simulink model "Sensors_and_actuators_ball_and_plate"  (R2022b)
settings: Solver=ode1  StartTime=0.0  StopTime=Inf  FixedStep=0.001  RelTol=1e-3
PostLoadFcn:
  | , if any(exist('dsrtsu_mdlpostloadfcn', 'file') ~= 0), dsrtsu_mdlpostloadfcn('Execute', bdroot); end,
InitFcn:
  | , if any(exist('rtifpga_mdlclblib', 'file') ~= 0), rtifpga_mdlclblib('Init', bdroot); end,
values from neighbouring files (symbols this model uses):
  denc_mi = C.Denominator{:}    [main.m]
  numc_mi = C.Numerator{:}    [main.m]
libraries: rtiemclib x6, rtiethernetlib x3, rti1202lib_dac_class1 x3
(part 2 of 2)

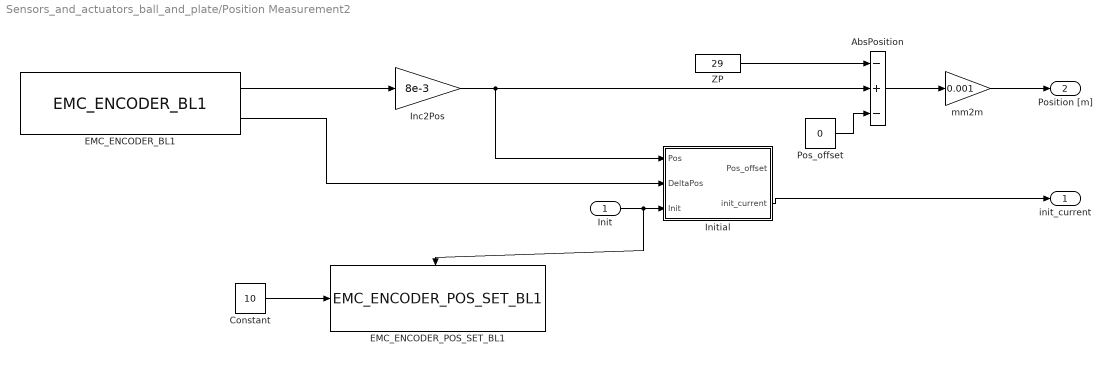
== system Sensors_and_actuators_ball_and_plate/Position Measurement2 ==
  Init : Inport
  AbsPosition : Sum  Inputs=-+-  SaturateOnIntegerOverflow=on
  Constant : Constant  Value=10
  EMC_ENCODER_BL1 : rtiemclib/EMC_ENCODER_BL1  DSProperties=struct('RTI',struct('Version',uint32(2),'BlockType',struct('isSLSource',uint8(1),'isSLSink',uint8(0),'isHWSource',uint8(1),'isHWSink',uint8(0),'isSetup',uint8(0),'isInline',uint8(1),'isNonInline',uint8(0),'isInterrupt',uint8(0),'isChannelwise',uint8(1)),'IOBoardType','DSEMC','UnitType','ENCODER','Identifier','ENCODER','DialogType','ML','BlockSet','RTIEMC','SlaveProcessor','NONE'))  RTIBlockInterface=struct('OutputPortsWidth',int32([1 1 1]),'OutputPortsActive',int32([1 1 0]),'OutputPortsName',{{'Position','Speed',['Index Detected']}},'OutputPortsDataType',{{'SS_DOUBLE','SS_DOUBLE','SS_BOOLEAN'}},'InitLevel',3,'IconTransparency','on','BlockDisplay',{{['EMC Encoder\nUnit: 3\nDIO class: 2\nPort: 1\nChannel: 5'],'center'}},'DialogFcn','rtiemcencodergui','BlockName',struct('Token',{{'EMC_ENCODER_BL1'}}))  RTIBlockParameters=struct('UnitNo',{{3,'OFF',[1 6]}},'DioClassNo',{{2,'OFF',[1 2]}},'PortNo',{{1,'OFF',[1 1]}},'ChannelNo',{{5,'OFF',[1 11]}},'HwSignalPin',{{['DIO1 ch1'],'OFF',[]}},'HwRefPin',{{'GND','OFF',[]}},'EnablePosMeasurement',{{1,'OFF',[0 1]}},'IndexSetMode',{{1,'OFF',[1 3]}},'EnableMinSpeed',{{0,'OFF',[0 1]}},'NumOfLines',{{'1024','OFF',[1 2097152]}},'InitAngleValue',{{'60','OFF',[0 359.99999]}},'IndexAngleValue',{{'0','OFF',[0 359.99999]}},'MinSpeedAngleValue',{{'45','OFF',[0.05 10000]}},'MinPosValue',{{'0','OFF',[-2097152 2097150.75]}},'MaxPosValue',{{'10000','OFF',[-2097151 2097151.75]}},'InitPosValue',{{'0','OFF',[-2097152 2097151.75]}},'IndexPosValue',{{'0','OFF',[-2097152 2097151.75]}},'MinSpeedPosValue',{{'100','OFF',[1 1000000]}},'IndexGateMode',{{0,'OFF',[0 1]}},'EnableNoiseFilter',{{0,'OFF',[0 1]}},'FilterInterval',{{'0','OFF',[0 0.01]}},'IndexDetectedOutPortMode',{{0,'OFF',[0 1]}},'BuildCheckAngleMeasurement',{{0,'OFF',[0 1]}},'BuildCheckAngleIndexMode',{{0,'OFF',[0 1]}},'BuildCheckPosIndexMode',{{0,'OFF',[0 1]}},'BuildCheckAngleMinSpeed',{{0,'OFF',[0 1]}},'BuildCheckPosMinSpeed',{{0,'OFF',[0 1]}},'TLCFileName',{{'rtiemcencoder','OFF',[]}})  RTISFcnParameters=struct('UnitNo','int32','DioClassNo','int32','PortNo','int32','ChannelNo','int32','EnablePosMeasurement','int32','IndexSetMode','int32','IndexDetectedOutPortMode','int32','EnableMinSpeed','int32','NumOfLines','uint32','InitAngleValue','double','IndexAngleValue','double','MinSpeedAngleValue','double','MinPosValue','double','MaxPosValue','double','InitPosValue','double','IndexPosValue','double','MinSpeedPosValue','double','IndexGateMode','int32','EnableNoiseFilter','int32','FilterInterval','double','TLCFileName','char')  RTIBlockParaDefault=struct('UnitNo',1,'DioClassNo',1,'PortNo',1,'ChannelNo',1,'HwSignalPin',['DIO1 ch1'],'HwRefPin','GND','EnablePosMeasurement',0,'IndexSetMode',1,'EnableMinSpeed',0,'NumOfLines',1024,'InitAngleValue',60,'IndexAngleValue',0,'MinSpeedAngleValue',45,'MinPosValue',0,'MaxPosValue',1023.75,'InitPosValue',0,'IndexPosValue',0,'MinSpeedPosValue',100,'IndexGateMode',0,'EnableNoiseFilter',0,'FilterInterval',0,'IndexDetectedOutPortMode',0,'BuildCheckAngleMeasurement',1,'BuildCheckAngleIndexMode',0,'BuildCheckPosIndexMode',0,'BuildCheckAngleMinSpeed',0,'BuildCheckPosMinSpeed',0,'TLCFileName','rtiemcencoder')
  EMC_ENCODER_POS_SET_BL1 : rtiemclib/EMC_ENCODER_POS_SET_BL1  DSProperties=struct('RTI',struct('Version',uint32(1),'BlockType',struct('isSLSource',uint8(0),'isSLSink',uint8(1),'isHWSource',uint8(0),'isHWSink',uint8(1),'isSetup',uint8(0),'isInline',uint8(1),'isNonInline',uint8(0),'isInterrupt',uint8(0),'isChannelwise',uint8(1)),'IOBoardType','DSEMC','UnitType','ENCODER','Identifier','ENCODERPOSSET','DialogType','ML','BlockSet','RTIEMC','SlaveProcessor','NONE'))  RTIBlockInterface=struct('InputPortsWidth',int32(1),'InputPortsActive',1,'InputPortsDataType',{{'SS_DOUBLE'}},'InputPortsName',{{'Position'}},'TriggerPort',{{'rising'}},'InitLevel',3,'IconTransparency','on','BlockDisplay',{{['EMC Encoder Position Set\nUnit: 3\nDIO class: 2\nPort: 1\nChannel: 5'],'center'}},'DialogFcn','rtiemcencoderpossetgui','BlockName',struct('Token',{{'EMC_ENCODER_POS_SET_BL1'}}))  RTIBlockParameters=struct('EncoderIdIndex',{{4,'OFF',[1 4]}},'UnitNo',{{3,'OFF',[]}},'DioClassNo',{{2,'OFF',[]}},'PortNo',{{1,'OFF',[]}},'ChannelNo',{{5,'OFF',[]}},'EnablePosMeasurement',{{1,'OFF',[]}},'NumOfLines',{{1024,'OFF',[]}},'TLCFileName',{{'rtiemcencoderposset','OFF',[]}})  RTISFcnParameters=struct('EncoderIdIndex','int32','UnitNo','int32','DioClassNo','int32','PortNo','int32','ChannelNo','int32','EnablePosMeasurement','int32','NumOfLines','int32','TLCFileName','char')  RTIBlockParaDefault=struct('EncoderIdIndex',1,'UnitNo',-1,'DioClassNo',-1,'PortNo',-1,'ChannelNo',-1,'EnablePosMeasurement',0,'NumOfLines',1024,'TLCFileName','rtiemcencoderposset')
  Inc2Pos : Gain  Gain=8e-3  SaturateOnIntegerOverflow=on  OutDataTypeStr=Inherit: Same as input  ParamDataTypeStr=Inherit: Same as input
  Initial : Subsystem
  Pos_offset : Constant  Value=0
  ZP : Constant  Value=29
  mm2m : Gain  Gain=0.001
  init_current : Outport  VectorParamsAs1DForOutWhenUnconnected=off
  Position [m] : Outport  Port=2  VectorParamsAs1DForOutWhenUnconnected=off
  wires:
  AbsPosition/1 -> mm2m/1
  Inc2Pos/1 -> Initial/1(Pos), AbsPosition/2
  Initial/2(init_current) -> init_current/1
  mm2m/1 -> Position [m]/1
  EMC_ENCODER_BL1/2 -> Initial/2(DeltaPos)
  ZP/1 -> AbsPosition/1
  Constant/1 -> EMC_ENCODER_POS_SET_BL1/1
  Init/1 -> Initial/3(Init), EMC_ENCODER_POS_SET_BL1/Trigger
  Pos_offset/1 -> AbsPosition/3
  EMC_ENCODER_BL1/1 -> Inc2Pos/1

== system Sensors_and_actuators_ball_and_plate/RTI Data ==
  RTI Data Store : Subsystem  Tag="struct('private',struct('version',struct('dsVer',uint32(2)),'access',struct('modified',['16-May-2023 15:23:02'],'type','Model','isPerm',1)),'public',struct('main',struct('data',[]),'sub',struct('name',{{'Sensors_and_actuators_ball_and_plate'}},'data',{{struct('TH',struct('thTaskInfo',struct('taskType',{'TIMER','HWINT','TMRINT','SWINT','GLINT'},'tasksNumOf',{1,0,0,0,0},'srcIds',{{'TIMERA'},{},{},{},{}},'taskNames',{{['Timer Task 1']},{},{},{},{}})),'th_tc',struct('dataType','TASK','taskGroupId','','taskGroupList',{{}},'taskSchedulingPolicy','FCFS','taskType','TIMER','blkh',-1,'srcId','TIMERA','srcSgnName',['Timer A interrupt'],'srcCpuName','','taskName',['Timer Task 1  [0.001] s'],'taskNameDisplayExt','','smplTime',0.001,'smplTimeOffs',0,'hasFixedPriority',0,'priority',1,'hasFixedOvc',0,'ovcType',1,'ovcMax',1),'tc_th',struct('dataType','TASK','taskGroupId','','taskGroupList',{{}},'taskSchedulingPolicy','FCFS','taskType','TIMER','blkh',-1,'srcId','TIMERA','srcSgnName',['Timer A interrupt'],'srcCpuName','','taskName',['Timer Task 1  [0.001] s'],'taskNameDisplayExt','','smplTime',0.001,'smplTimeOffs',0,'hasFixedPriority',0,'priority',1,'hasFixedOvc',0,'ovcType',1,'ovcMax',1))}})))"  mask(RTI_DATA_STORE){}
      mask help:
      | RTI Data Store Block. This block is used by RTI to store internal model dependent data. Deleting this block will result in data loss.
      |
      | NEVER DELETE, COPY, OR MODIFY THIS BLOCK!
      mask Help:
      | RTI Data Store Block. This block is used by RTI to store internal model dependent data. Deleting this block will result in data loss.
      | 
      | NEVER DELETE, COPY, OR MODIFY THIS BLOCK!
      mask Display: text(0.5, 0.5, ' ', 'HorizontalAlignment', 'center');

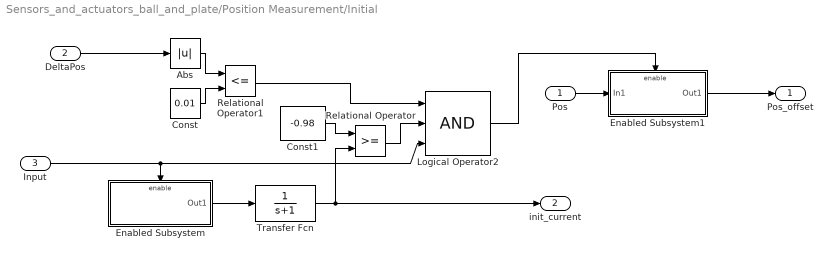
== system Sensors_and_actuators_ball_and_plate/Position Measurement/Initial ==
  Pos : Inport
  DeltaPos : Inport  Port=2
  Input : Inport  Port=3
  Abs : Abs
  Const : Constant  Value=0.01
  Const1 : Constant  Value=-0.98
  Enabled Subsystem : Subsystem  TreatAsAtomicUnit=on
  Enabled Subsystem1 : Subsystem  TreatAsAtomicUnit=on
  Logical Operator2 : Logic  Inputs=3  AllPortsSameDT=off
  Relational Operator : RelationalOperator  InputSameDT=off
  Relational Operator1 : RelationalOperator  Operator=<=  InputSameDT=off
  Transfer Fcn : TransferFcn  Denominator=[1 1]
  Pos_offset : Outport  VectorParamsAs1DForOutWhenUnconnected=off
  init_current : Outport  Port=2  VectorParamsAs1DForOutWhenUnconnected=off
  wires:
  Enabled Subsystem/1(Out1) -> Transfer Fcn/1
  Transfer Fcn/1 -> Relational Operator/2, init_current/1
  Input/1 -> Enabled Subsystem/Enable, Logical Operator2/3
  Const1/1 -> Relational Operator/1
  Abs/1 -> Relational Operator1/1
  Const/1 -> Relational Operator1/2
  Relational Operator1/1 -> Logical Operator2/1
  Relational Operator/1 -> Logical Operator2/2
  DeltaPos/1 -> Abs/1
  Logical Operator2/1 -> Enabled Subsystem1/Enable
  Pos/1 -> Enabled Subsystem1/1(In1)
  Enabled Subsystem1/1(Out1) -> Pos_offset/1

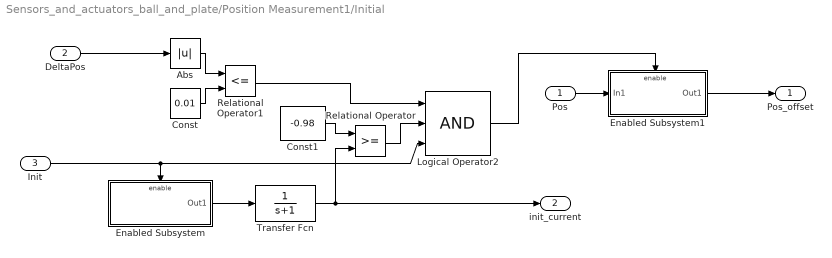
== system Sensors_and_actuators_ball_and_plate/Position Measurement1/Initial ==
  Pos : Inport
  DeltaPos : Inport  Port=2
  Init : Inport  Port=3
  Abs : Abs
  Const : Constant  Value=0.01
  Const1 : Constant  Value=-0.98
  Enabled Subsystem : Subsystem  TreatAsAtomicUnit=on
  Enabled Subsystem1 : Subsystem  TreatAsAtomicUnit=on
  Logical Operator2 : Logic  Inputs=3  AllPortsSameDT=off
  Relational Operator : RelationalOperator  InputSameDT=off
  Relational Operator1 : RelationalOperator  Operator=<=  InputSameDT=off
  Transfer Fcn : TransferFcn  Denominator=[1 1]
  Pos_offset : Outport  VectorParamsAs1DForOutWhenUnconnected=off
  init_current : Outport  Port=2  VectorParamsAs1DForOutWhenUnconnected=off
  wires:
  Enabled Subsystem/1(Out1) -> Transfer Fcn/1
  Transfer Fcn/1 -> Relational Operator/2, init_current/1
  Init/1 -> Enabled Subsystem/Enable, Logical Operator2/3
  Const1/1 -> Relational Operator/1
  Abs/1 -> Relational Operator1/1
  Const/1 -> Relational Operator1/2
  Relational Operator1/1 -> Logical Operator2/1
  Relational Operator/1 -> Logical Operator2/2
  DeltaPos/1 -> Abs/1
  Logical Operator2/1 -> Enabled Subsystem1/Enable
  Pos/1 -> Enabled Subsystem1/1(In1)
  Enabled Subsystem1/1(Out1) -> Pos_offset/1

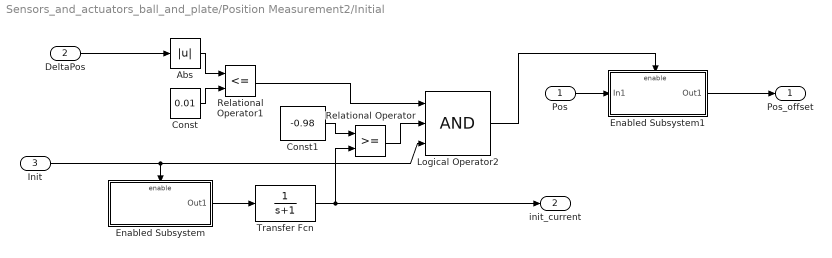
== system Sensors_and_actuators_ball_and_plate/Position Measurement2/Initial ==
  Pos : Inport
  DeltaPos : Inport  Port=2
  Init : Inport  Port=3
  Abs : Abs
  Const : Constant  Value=0.01
  Const1 : Constant  Value=-0.98
  Enabled Subsystem : Subsystem  TreatAsAtomicUnit=on
  Enabled Subsystem1 : Subsystem  TreatAsAtomicUnit=on
  Logical Operator2 : Logic  Inputs=3  AllPortsSameDT=off
  Relational Operator : RelationalOperator  InputSameDT=off
  Relational Operator1 : RelationalOperator  Operator=<=  InputSameDT=off
  Transfer Fcn : TransferFcn  Denominator=[1 1]
  Pos_offset : Outport  VectorParamsAs1DForOutWhenUnconnected=off
  init_current : Outport  Port=2  VectorParamsAs1DForOutWhenUnconnected=off
  wires:
  Enabled Subsystem/1(Out1) -> Transfer Fcn/1
  Transfer Fcn/1 -> Relational Operator/2, init_current/1
  Init/1 -> Enabled Subsystem/Enable, Logical Operator2/3
  Const1/1 -> Relational Operator/1
  Abs/1 -> Relational Operator1/1
  Const/1 -> Relational Operator1/2
  Relational Operator1/1 -> Logical Operator2/1
  Relational Operator/1 -> Logical Operator2/2
  DeltaPos/1 -> Abs/1
  Logical Operator2/1 -> Enabled Subsystem1/Enable
  Pos/1 -> Enabled Subsystem1/1(In1)
  Enabled Subsystem1/1(Out1) -> Pos_offset/1

== system Sensors_and_actuators_ball_and_plate/RTI Data/RTI Data Store ==
  RTI Data Store : Subsystem  mask(RTI_DATA_STORE){}
      mask help:
      | RTI Data Store Block. This block is used by RTI to store internal model dependent data. Deleting this block will result in data loss.
      |
      | NEVER DELETE, COPY, OR MODIFY THIS BLOCK!
      mask Help:
      | RTI Data Store Block. This block is used by RTI to store internal model dependent data. Deleting this block will result in data loss.
      | 
      | NEVER DELETE, COPY, OR MODIFY THIS BLOCK!
      mask Display: text(0.5, 0.5, ' ', 'HorizontalAlignment', 'center');

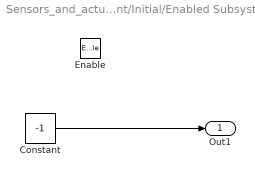
== system Sensors_and_actuators_ball_and_plate/Position Measurement/Initial/Enabled Subsystem ==
  Enable : EnablePort  PropagateVarSize=During execution
  Constant : Constant  Value=-1
  Out1 : Outport  OutputWhenDisabled=reset  InitialOutput=[0]  VectorParamsAs1DForOutWhenUnconnected=off
  wires:
  Constant/1 -> Out1/1

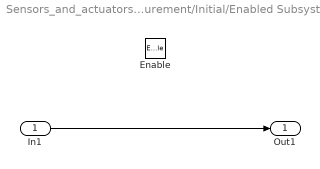
== system Sensors_and_actuators_ball_and_plate/Position Measurement/Initial/Enabled Subsystem1 ==
  In1 : Inport
  Enable : EnablePort  PropagateVarSize=During execution
  Out1 : Outport  InitialOutput=[0]  VectorParamsAs1DForOutWhenUnconnected=off
  wires:
  In1/1 -> Out1/1

== system Sensors_and_actuators_ball_and_plate/Position Measurement1/Initial/Enabled Subsystem ==
  Enable : EnablePort  PropagateVarSize=During execution
  Constant : Constant  Value=-1
  Out1 : Outport  OutputWhenDisabled=reset  InitialOutput=[0]  VectorParamsAs1DForOutWhenUnconnected=off
  wires:
  Constant/1 -> Out1/1

== system Sensors_and_actuators_ball_and_plate/Position Measurement1/Initial/Enabled Subsystem1 ==
  In1 : Inport
  Enable : EnablePort  PropagateVarSize=During execution
  Out1 : Outport  InitialOutput=[0]  VectorParamsAs1DForOutWhenUnconnected=off
  wires:
  In1/1 -> Out1/1

== system Sensors_and_actuators_ball_and_plate/Position Measurement2/Initial/Enabled Subsystem ==
  Enable : EnablePort  PropagateVarSize=During execution
  Constant : Constant  Value=-1
  Out1 : Outport  OutputWhenDisabled=reset  InitialOutput=[0]  VectorParamsAs1DForOutWhenUnconnected=off
  wires:
  Constant/1 -> Out1/1

== system Sensors_and_actuators_ball_and_plate/Position Measurement2/Initial/Enabled Subsystem1 ==
  In1 : Inport
  Enable : EnablePort  PropagateVarSize=During execution
  Out1 : Outport  InitialOutput=[0]  VectorParamsAs1DForOutWhenUnconnected=off
  wires:
  In1/1 -> Out1/1

== system Sensors_and_actuators_ball_and_plate/RTI Data/RTI Data Store/RTI Data Store ==
  RTI Data Store : Subsystem  mask(RTI_DATA_STORE){}
      mask help:
      | RTI Data Store Block. This block is used by RTI to store internal model dependent data. Deleting this block will result in data loss.
      |
      | NEVER DELETE, COPY, OR MODIFY THIS BLOCK!
      mask Help:
      | RTI Data Store Block. This block is used by RTI to store internal model dependent data. Deleting this block will result in data loss.
      | 
      | NEVER DELETE, COPY, OR MODIFY THIS BLOCK!
      mask Display: text(0.5, 0.5, ' ', 'HorizontalAlignment', 'center');

== system Sensors_and_actuators_ball_and_plate/RTI Data/RTI Data Store/RTI Data Store/RTI Data Store ==
  RTI Data Store : Subsystem  mask(RTI_DATA_STORE){}
      mask help:
      | RTI Data Store Block. This block is used by RTI to store internal model dependent data. Deleting this block will result in data loss.
      |
      | NEVER DELETE, COPY, OR MODIFY THIS BLOCK!
      mask Help:
      | RTI Data Store Block. This block is used by RTI to store internal model dependent data. Deleting this block will result in data loss.
      | 
      | NEVER DELETE, COPY, OR MODIFY THIS BLOCK!
      mask Display: text(0.5, 0.5, ' ', 'HorizontalAlignment', 'center');

== system Sensors_and_actuators_ball_and_plate/RTI Data/RTI Data Store/RTI Data Store/RTI Data Store/RTI Data Store ==
